simulink model "sf_gfdemo"  (Simulink 6.0)
settings: Solver=ode45  StartTime=0.0  StopTime=10  MaxStep=.01  RelTol=1e-3
settings Model: CovMetricSettings=dcmtr  Creator=The MathWorks Inc.  LastModifiedBy=batserve  ExtModeAutoUpdateStatusClock=off
settings OptimizationCC: BooleanDataType=off
settings DebuggingCC: CheckExecutionContextPreStartOutputMsg=on  CheckExecutionContextRuntimeOutputMsg=on  SolverPrmCheckMsg=none
settings HardwareCC: TargetUnknown=on

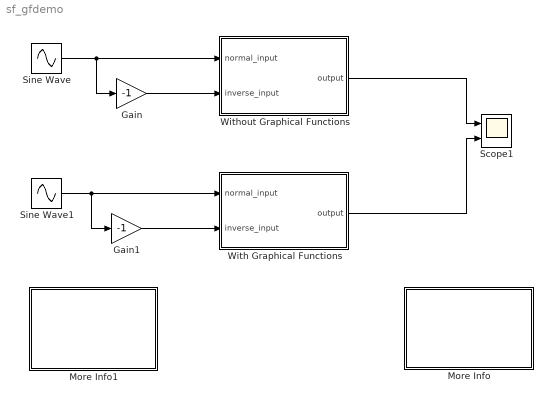
== system sf_gfdemo ==
  Gain : Gain  Gain=-1  SaturateOnIntegerOverflow=on
  Gain1 : Gain  Gain=-1  SaturateOnIntegerOverflow=on
  More Info : Subsystem  PropExecContextAcrossSSBoundary=on
      mask Display: disp('Double click\nhere for\ninformation on\nthis demonstration')
  More Info1 : Subsystem  PropExecContextAcrossSSBoundary=on
      settings: OpenFcn=simcad(bdroot);
      mask Display: disp('Double click\nhere for\nSimulink\Stateflow\n Help')
  Scope1 : Scope  NumInputPorts=2
      settings: TimeRange=10  YMin=-0.5~-0.5  YMax=1~1
  Sine Wave : Sin  SampleTime=0
  Sine Wave1 : Sin  SampleTime=0
  With Graphical Functions : Stateflow chart  PropExecContextAcrossSSBoundary=on
  Without Graphical Functions : Stateflow chart  PropExecContextAcrossSSBoundary=on
  wires:
  Without Graphical Functions/1(output) -> Scope1/1
  With Graphical Functions/1(output) -> Scope1/2
  Sine Wave/1 -> Gain/1, Without Graphical Functions/1(normal_input)
  Gain/1 -> Without Graphical Functions/2(inverse_input)
  Sine Wave1/1 -> Gain1/1, With Graphical Functions/1(normal_input)
  Gain1/1 -> With Graphical Functions/2(inverse_input)

== system sf_gfdemo/More Info ==
  note: Graphical Function Demonstration
  note: This demonstration shows the concept of a graphical function and how it can be used to simplify
      | your Stateflow model. In this example, we pass two inputs in the Stateflow chart. The first input is
      | a sine wave with magnitude 1 and a frequency of 2*pi and the second input is that same sine wave
      | but inverted. The Stateflow charts output only the positive values of both the input signals and also
      | saturate the signal at a value of 0.5.
      |
      | In the first chart, 'Without Graphical Functions', the output is defined directly within the substate. The
      | Normal state is activated first, and the output is set equal to the normal_input. When the
      | normal_input is greater than 0.5, the output is set equal to 0.5. When the normal_input becomes
      |  negative (<0), then a state transition occurs, and the output is redefined the same way within the
      |  Inverse state, except that the inverse_input is used.
      |
      | In the 'With Graphical Functions' chart, the output is defined by calling the graphical function. Instead
      | of defining the saturation transition (where the output remains at the 0.5 value) within the states, we
      | only define it once in the graphical function. Although it is not as evident in this simple demo, when
      | more conditions and parameters are introduced, and the output needs to be defined in multiple
      | states, graphical functions allow you to simplify your model.

== system sf_gfdemo/More Info1 ==

== stateflow chart Without Graphical Functions ==
  state Normal
    (default) -> (junction 5)
    (junction 5) -> (junction 9) : [normal_input >0.5]
    (junction 9) -> (junction 10) : {output = 0.5;}
    (junction 5) -> (junction 10) : {output=normal_input;}
  state Inverse
    (default) -> (junction 6)
    (junction 6) -> (junction 7) : [inverse_input > 0.5]
    (junction 6) -> (junction 8) : {output=inverse_input;}
    (junction 7) -> (junction 8) : {output = 0.5;}
  (default) -> Normal
  Normal -> Inverse : [normal_input < 0]
  Inverse -> Normal : [inverse_input<0]
  Normal -> Normal
  Inverse -> Inverse
  data: output output double; normal_input input double; inverse_input input double
  events: Switch local EITHER_EDGE_EVENT

== stateflow chart With Graphical Functions ==
  settings: updateMethod=CONTINUOUS
  state Normal
    (default) -> (junction 34) : {set_output_data(normal_input);}
  state Inverse
    (default) -> (junction 35) : {set_output_data(inverse_input);}
  state set_output_data(input) [function]
    (default) -> (junction 33)
    (junction 33) -> (junction 36) : [input>.5]
    (junction 36) -> (junction 37) : {output = 0.5;}
    (junction 33) -> (junction 37) : {output = input;}
  (default) -> Normal
  Normal -> Inverse : [normal_input < 0]
  Inverse -> Normal : [inverse_input<0]
  Normal -> Normal
  Inverse -> Inverse
  data: input function_input double; output output double; normal_input input double; inverse_input input double
